simulink model "Buck_DCM_Due"  (R2020a)
settings: Solver=FixedStepAuto  StartTime=0.0  StopTime=10  FixedStep=T  RelTol=1e-3  EnableMultiTasking=on
undefined symbols (not defined in the file): C, ILmax, Iumax, J, Ki_I, Ki_IL, Kp_I, Kp_IL, Kp_Uc, Kp_W, Kphi, L, Lu, rL, Ru, T, Ubat, Ucmax, wmax
libraries: arduinolib x20, simulink x16
(part 1 of 2)
settings Model: SILPILModeSetting=veronly  ExtModeTrigDuration=2  Creator=Nguyen Tung  LastModifiedBy=Nguyen Tung
settings SolverCC: PositivePriorityOrder=on
settings OptimizationCC: StrengthReduction=on  PassReuseOutputArgsAs=Individual arguments  ZeroExternalMemoryAtStartup=off  ZeroInternalMemoryAtStartup=off  MaxStackSize=64  OptimizeBlockOrder=speed  OptimizationPriority=Speed  OptimizationCustomize=off  MultiThreadedLoops=on  EfficientTunableParamExpr=on
settings DebuggingCC: ParameterTunabilityLossMsg=error
settings HardwareCC: ProdBitPerPointer=32  ProdBitPerSizeT=32  ProdBitPerPtrDiffT=32  ProdLargestAtomicInteger=Long  ProdLargestAtomicFloat=Double  ProdWordSize=32  ProdHWDeviceType=ARM Compatible->ARM Cortex
settings SFSimCC: MATLABDynamicMemAlloc=off
settings RTWCC: SystemTargetFile=ert.tlc  HardwareBoard=Arduino Due  TLCOptions="-aInlineSetEventsForThisBaseRateFcn=TLC_FALSE -aSuppressMultiTaskScheduler=TLC_FALSE   -aRateBasedStepFcn=1"  TemplateMakefile=ert_default_tmf  Toolchain=Arduino ARM  BuildConfiguration=Faster Runs
settings CodeAppCC: ForceParamTrailComments=on  IgnoreCustomStorageClasses=off  OperatorAnnotations=on  SimulinkDataObjDesc=on  SFDataObjDesc=on  InsertBlockDesc=on
settings ERTTargetCC: SupportContinuousTime=on  SupportVariableSizeSignals=on  ExtModeStaticAllocSize=24576

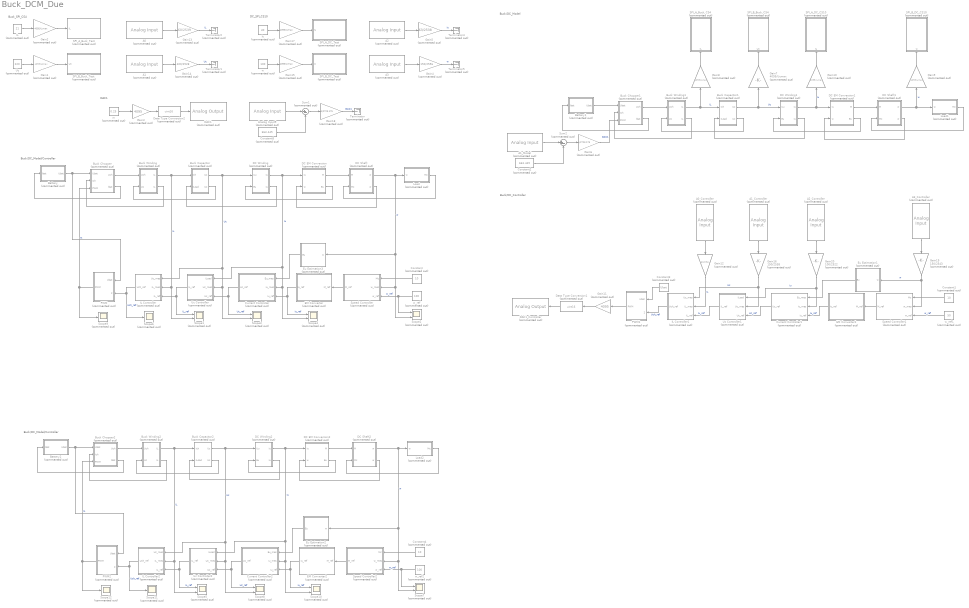
== system Buck_DCM_Due ==
  note: Buck/DC_Controller
  note: Buck/DC_Model
  note: Buck/DC_Model/Controller
  note: DAC1
  note: Buck_SPI_CS4
  note: DC_SPI_CS10
  note: Buck/DC_Model/Controller
  A0 : arduinolib/Analog Input  Commented=on  pinNumber=0  ReadResultsOnly=off  ConversionTriggerSource=Software  ExternalTriggerType=uint32( 0 )  OutputDataType=uint16  EnableConversionCompleteNotify=off  EnableOuputStatus=off  SampleTime=T  blockPlatform=arduino
  A0_Controller : arduinolib/Analog Input  Commented=on  pinNumber=0  ReadResultsOnly=off  ConversionTriggerSource=Software  ExternalTriggerType=uint32( 0 )  OutputDataType=uint16  EnableConversionCompleteNotify=off  EnableOuputStatus=off  SampleTime=T  blockPlatform=arduino
  A1 : arduinolib/Analog Input  Commented=on  pinNumber=1  ReadResultsOnly=off  ConversionTriggerSource=Software  ExternalTriggerType=uint32( 0 )  OutputDataType=uint16  EnableConversionCompleteNotify=off  EnableOuputStatus=off  SampleTime=T  blockPlatform=arduino
  A1_Controller : arduinolib/Analog Input  Commented=on  pinNumber=1  ReadResultsOnly=off  ConversionTriggerSource=Software  ExternalTriggerType=uint32( 0 )  OutputDataType=uint16  EnableConversionCompleteNotify=off  EnableOuputStatus=off  SampleTime=T  blockPlatform=arduino
  A1_Model : arduinolib/Analog Input  Commented=on  pinNumber=1  ReadResultsOnly=off  ConversionTriggerSource=Software  ExternalTriggerType=uint32( 0 )  OutputDataType=uint16  EnableConversionCompleteNotify=off  EnableOuputStatus=off  SampleTime=T  blockPlatform=arduino
  A2 : arduinolib/Analog Input  Commented=on  pinNumber=2  ReadResultsOnly=off  ConversionTriggerSource=Software  ExternalTriggerType=uint32( 0 )  OutputDataType=uint16  EnableConversionCompleteNotify=off  EnableOuputStatus=off  SampleTime=T  blockPlatform=arduino
  A2_Controller : arduinolib/Analog Input  Commented=on  pinNumber=2  ReadResultsOnly=off  ConversionTriggerSource=Software  ExternalTriggerType=uint32( 0 )  OutputDataType=uint16  EnableConversionCompleteNotify=off  EnableOuputStatus=off  SampleTime=T  blockPlatform=arduino
  A3 : arduinolib/Analog Input  Commented=on  pinNumber=3  ReadResultsOnly=off  ConversionTriggerSource=Software  ExternalTriggerType=uint32( 0 )  OutputDataType=uint16  EnableConversionCompleteNotify=off  EnableOuputStatus=off  SampleTime=T  blockPlatform=arduino
  A3_Controller : arduinolib/Analog Input  Commented=on  pinNumber=3  ReadResultsOnly=off  ConversionTriggerSource=Software  ExternalTriggerType=uint32( 0 )  OutputDataType=uint16  EnableConversionCompleteNotify=off  EnableOuputStatus=off  SampleTime=T  blockPlatform=arduino
  Analog Input9 : arduinolib/Analog Input  Commented=on  pinNumber=1  ReadResultsOnly=off  ConversionTriggerSource=Software  ExternalTriggerType=uint32( 0 )  OutputDataType=uint16  EnableConversionCompleteNotify=off  EnableOuputStatus=off  SampleTime=T  blockPlatform=arduino
  Battery : Subsystem  Commented=on  AncestorBlock=simulink/REM/SE
      mask Display:
      | plot(0,0,100,100, 1.2*[50,57.68,60.77,63.08,64.97,66.58,68,69.26,70.4, 	71.42,72.36,78.28,80,78.28,72.36,71.42,70.4, 	69.26,68,66.58,64.97,63.08,60.77,57.68,50,42.32, 	39.23,36.92,35.03,33.42,32,30.74,29.6,28.58, 	27.64,21.72,20,21.72,27.64,28.58,29.6,30.74,32, 	33.42,35.03,36.92,39.23,42.32,50]-10, 1.2*[20,21,22,23,24,25,26,27,28,29,30,40,50,60,70,71,72, 	73,74,75,76,77,78,79,80,79,78,77,76,75,74,73,72, 	71,70,60,50,40,30,29,28,27,26,25,24,23,22,21,20]-10)
      | disp('ES')
  Battery1 : Subsystem  Commented=on  AncestorBlock=simulink/REM/SE
      mask Display:
      | plot(0,0,100,100, 1.2*[50,57.68,60.77,63.08,64.97,66.58,68,69.26,70.4, 	71.42,72.36,78.28,80,78.28,72.36,71.42,70.4, 	69.26,68,66.58,64.97,63.08,60.77,57.68,50,42.32, 	39.23,36.92,35.03,33.42,32,30.74,29.6,28.58, 	27.64,21.72,20,21.72,27.64,28.58,29.6,30.74,32, 	33.42,35.03,36.92,39.23,42.32,50]-10, 1.2*[20,21,22,23,24,25,26,27,28,29,30,40,50,60,70,71,72, 	73,74,75,76,77,78,79,80,79,78,77,76,75,74,73,72, 	71,70,60,50,40,30,29,28,27,26,25,24,23,22,21,20]-10)
      | disp('ES')
  Battery2 : Subsystem  Commented=on  AncestorBlock=simulink/REM/SE
      mask Display:
      | plot(0,0,100,100, 1.2*[50,57.68,60.77,63.08,64.97,66.58,68,69.26,70.4, 	71.42,72.36,78.28,80,78.28,72.36,71.42,70.4, 	69.26,68,66.58,64.97,63.08,60.77,57.68,50,42.32, 	39.23,36.92,35.03,33.42,32,30.74,29.6,28.58, 	27.64,21.72,20,21.72,27.64,28.58,29.6,30.74,32, 	33.42,35.03,36.92,39.23,42.32,50]-10, 1.2*[20,21,22,23,24,25,26,27,28,29,30,40,50,60,70,71,72, 	73,74,75,76,77,78,79,80,79,78,77,76,75,74,73,72, 	71,70,60,50,40,30,29,28,27,26,25,24,23,22,21,20]-10)
      | disp('ES')
  Buck Capacitor : Subsystem  Commented=on  AncestorBlock=simulink/REM/EA  mask(CM){}
      mask Display: plot(0,0,100,100,[10,10,90,90,10],[90,10,10,90,90], [10,90],[10,90])
  Buck Capacitor1 : Subsystem  Commented=on  AncestorBlock=simulink/REM/EA  mask(CM){}
      mask Display: plot(0,0,100,100,[10,10,90,90,10],[90,10,10,90,90], [10,90],[10,90])
  Buck Capacitor2 : Subsystem  Commented=on  AncestorBlock=simulink/REM/EA  mask(CM){}
      mask Display: plot(0,0,100,100,[10,10,90,90,10],[90,10,10,90,90], [10,90],[10,90])
  Buck Chopper : Subsystem  Commented=on  AncestorBlock=simulink/REM/EC Elec  mask(Hacheur){}
      mask Display: plot(0,0,100,100,[10,10,90,90,10],[90,10,10,90,90])
  Buck Chopper1 : Subsystem  Commented=on  AncestorBlock=simulink/REM/EC Elec  mask(Hacheur){}
      mask Display: plot(0,0,100,100,[10,10,90,90,10],[90,10,10,90,90])
  Buck Chopper2 : Subsystem  Commented=on  AncestorBlock=simulink/REM/EC Elec  mask(Hacheur){}
      mask Display: plot(0,0,100,100,[10,10,90,90,10],[90,10,10,90,90])
  Buck Winding : Subsystem  Commented=on  AncestorBlock=simulink/REM/EA  mask(CM){}
      mask Display: plot(0,0,100,100,[10,10,90,90,10],[90,10,10,90,90], [10,90],[10,90])
  Buck Winding1 : Subsystem  Commented=on  AncestorBlock=simulink/REM/EA  mask(CM){}
      mask Display: plot(0,0,100,100,[10,10,90,90,10],[90,10,10,90,90], [10,90],[10,90])
  Buck Winding2 : Subsystem  Commented=on  AncestorBlock=simulink/REM/EA  mask(CM){}
      mask Display: plot(0,0,100,100,[10,10,90,90,10],[90,10,10,90,90], [10,90],[10,90])
  Constant : Constant  Commented=on  Value=10
  Constant1 : Constant  Commented=on  Value=10
  Constant2 : Constant  Commented=on  Value=663.445
  Constant3 : Constant  Commented=on  Value=Ubat
  Constant4 : Constant  Commented=on  Value=10
  Constant8 : Constant  Commented=on  Value=663.445
  Current Controller : Subsystem  Commented=on  AncestorBlock=simulink/SMC/Asservissement Correcteur IP
      mask Display: plot(0,0,100,100, [10,30,90,70,10,90],[90,10,10,90,90,10])
  Current Controller1 : Subsystem  Commented=on  AncestorBlock=simulink/SMC/Asservissement Correcteur IP
      mask Display: plot(0,0,100,100, [10,30,90,70,10,90],[90,10,10,90,90,10])
  Current Controller2 : Subsystem  Commented=on  AncestorBlock=simulink/SMC/Asservissement Correcteur IP
      mask Display: plot(0,0,100,100, [10,30,90,70,10,90],[90,10,10,90,90,10])
  DAC1 : arduinolib/Analog Output  Commented=on  DACpin=DAC1  blockPlatform=arduino
      settings: SourceProductBaseCode=ARDUINO
  DAC1_Controller : arduinolib/Analog Output  Commented=on  DACpin=DAC1  blockPlatform=arduino
      settings: SourceProductBaseCode=ARDUINO
  DC EM Conversion : Subsystem  Commented=on  AncestorBlock=simulink/REM/EC EM
      mask Display: plot(0,0,100,100, 1.4*[50,57.68,60.77,63.08,64.97,66.58,68,69.26,70.4, 	71.42,72.36,78.28,80,78.28,72.36,71.42,70.4, 	69.26,68,66.58,64.97,63.08,60.77,57.68,50,42.32, 	39.23,36.92,35.03,33.42,32,30.74,29.6,28.58, 	27.64,21.72,20,21.72,27.64,28.58,29.6,30.74,32, 	33.42,35.03,36.92,39.23,42.32,50]-20, 1.4*[20,21,22,23,24,25,26,27,28,29,30,40,50,60,70,71,72, 	73,74,75,76,77,78,79,80,79,78,77,76,75,74,73,72, 	71,70,60,50,40,30,29,28,27,26,25,24,23,22,21,20]-20)
  DC EM Conversion1 : Subsystem  Commented=on  AncestorBlock=simulink/REM/EC EM
      mask Display: plot(0,0,100,100, 1.4*[50,57.68,60.77,63.08,64.97,66.58,68,69.26,70.4, 	71.42,72.36,78.28,80,78.28,72.36,71.42,70.4, 	69.26,68,66.58,64.97,63.08,60.77,57.68,50,42.32, 	39.23,36.92,35.03,33.42,32,30.74,29.6,28.58, 	27.64,21.72,20,21.72,27.64,28.58,29.6,30.74,32, 	33.42,35.03,36.92,39.23,42.32,50]-20, 1.4*[20,21,22,23,24,25,26,27,28,29,30,40,50,60,70,71,72, 	73,74,75,76,77,78,79,80,79,78,77,76,75,74,73,72, 	71,70,60,50,40,30,29,28,27,26,25,24,23,22,21,20]-20)
  DC EM Conversion2 : Subsystem  Commented=on  AncestorBlock=simulink/REM/EC EM
      mask Display: plot(0,0,100,100, 1.4*[50,57.68,60.77,63.08,64.97,66.58,68,69.26,70.4, 	71.42,72.36,78.28,80,78.28,72.36,71.42,70.4, 	69.26,68,66.58,64.97,63.08,60.77,57.68,50,42.32, 	39.23,36.92,35.03,33.42,32,30.74,29.6,28.58, 	27.64,21.72,20,21.72,27.64,28.58,29.6,30.74,32, 	33.42,35.03,36.92,39.23,42.32,50]-20, 1.4*[20,21,22,23,24,25,26,27,28,29,30,40,50,60,70,71,72, 	73,74,75,76,77,78,79,80,79,78,77,76,75,74,73,72, 	71,70,60,50,40,30,29,28,27,26,25,24,23,22,21,20]-20)
  DC Shaft : Subsystem  Commented=on  AncestorBlock=simulink/REM/EA  mask(CM){}
      mask Display: plot(0,0,100,100,[10,10,90,90,10],[90,10,10,90,90], [10,90],[10,90])
  DC Shaft1 : Subsystem  Commented=on  AncestorBlock=simulink/REM/EA  mask(CM){}
      mask Display: plot(0,0,100,100,[10,10,90,90,10],[90,10,10,90,90], [10,90],[10,90])
  DC Shaft2 : Subsystem  Commented=on  AncestorBlock=simulink/REM/EA  mask(CM){}
      mask Display: plot(0,0,100,100,[10,10,90,90,10],[90,10,10,90,90], [10,90],[10,90])
  DC Winding : Subsystem  Commented=on  AncestorBlock=simulink/REM/EA  mask(CM){}
      mask Display: plot(0,0,100,100,[10,10,90,90,10],[90,10,10,90,90], [10,90],[10,90])
  DC Winding1 : Subsystem  Commented=on  AncestorBlock=simulink/REM/EA  mask(CM){}
      mask Display: plot(0,0,100,100,[10,10,90,90,10],[90,10,10,90,90], [10,90],[10,90])
  DC Winding2 : Subsystem  Commented=on  AncestorBlock=simulink/REM/EA  mask(CM){}
      mask Display: plot(0,0,100,100,[10,10,90,90,10],[90,10,10,90,90], [10,90],[10,90])
  Data Type Conversion1 : DataTypeConversion  Commented=on  OutDataTypeStr=uint16  RndMeth=Nearest
  Data Type Conversion2 : DataTypeConversion  Commented=on  OutDataTypeStr=uint16  RndMeth=Nearest
  EM Converter : Subsystem  Commented=on  AncestorBlock=simulink/SMC/Inversion EC avec mesure
      mask Display: plot(0,0,100,100,[10,30,90,70,10],[90,10,10,90,90])
  EM Converter1 : Subsystem  Commented=on  AncestorBlock=simulink/SMC/Inversion EC avec mesure
      mask Display: plot(0,0,100,100,[10,30,90,70,10],[90,10,10,90,90])
  EM Converter2 : Subsystem  Commented=on  AncestorBlock=simulink/SMC/Inversion EC avec mesure
      mask Display: plot(0,0,100,100,[10,30,90,70,10],[90,10,10,90,90])
  Eu Estimation1 : Subsystem  Commented=on  AncestorBlock=simulink/REM/EC EM
      mask Display: plot(0,0,100,100, 1.4*[50,57.68,60.77,63.08,64.97,66.58,68,69.26,70.4, 	71.42,72.36,78.28,80,78.28,72.36,71.42,70.4, 	69.26,68,66.58,64.97,63.08,60.77,57.68,50,42.32, 	39.23,36.92,35.03,33.42,32,30.74,29.6,28.58, 	27.64,21.72,20,21.72,27.64,28.58,29.6,30.74,32, 	33.42,35.03,36.92,39.23,42.32,50]-20, 1.4*[20,21,22,23,24,25,26,27,28,29,30,40,50,60,70,71,72, 	73,74,75,76,77,78,79,80,79,78,77,76,75,74,73,72, 	71,70,60,50,40,30,29,28,27,26,25,24,23,22,21,20]-20)
  Eu Estimation2 : Subsystem  Commented=on  AncestorBlock=simulink/REM/EC EM
      mask Display: plot(0,0,100,100, 1.4*[50,57.68,60.77,63.08,64.97,66.58,68,69.26,70.4, 	71.42,72.36,78.28,80,78.28,72.36,71.42,70.4, 	69.26,68,66.58,64.97,63.08,60.77,57.68,50,42.32, 	39.23,36.92,35.03,33.42,32,30.74,29.6,28.58, 	27.64,21.72,20,21.72,27.64,28.58,29.6,30.74,32, 	33.42,35.03,36.92,39.23,42.32,50]-20, 1.4*[20,21,22,23,24,25,26,27,28,29,30,40,50,60,70,71,72, 	73,74,75,76,77,78,79,80,79,78,77,76,75,74,73,72, 	71,70,60,50,40,30,29,28,27,26,25,24,23,22,21,20]-20)
  Eu Estimation3 : Subsystem  Commented=on  AncestorBlock=simulink/REM/EC EM
      mask Display: plot(0,0,100,100, 1.4*[50,57.68,60.77,63.08,64.97,66.58,68,69.26,70.4, 	71.42,72.36,78.28,80,78.28,72.36,71.42,70.4, 	69.26,68,66.58,64.97,63.08,60.77,57.68,50,42.32, 	39.23,36.92,35.03,33.42,32,30.74,29.6,28.58, 	27.64,21.72,20,21.72,27.64,28.58,29.6,30.74,32, 	33.42,35.03,36.92,39.23,42.32,50]-20, 1.4*[20,21,22,23,24,25,26,27,28,29,30,40,50,60,70,71,72, 	73,74,75,76,77,78,79,80,79,78,77,76,75,74,73,72, 	71,70,60,50,40,30,29,28,27,26,25,24,23,22,21,20]-20)
  Gain1 : Gain  Commented=on  Gain=4095/Ucmax
  Gain10 : Gain  Commented=on  Gain=4095/Iumax
  Gain11 : Gain  Commented=on  Gain=4095
  Gain12 : Gain  Commented=on  Gain=60/2541
  Gain13 : Gain  Commented=on  Gain=60/2539
  Gain14 : Gain  Commented=on  Gain=400/2528
  Gain15 : Gain  Commented=on  Gain=4095/wmax
  Gain16 : Gain  Commented=on  Gain=150/2538
  Gain17 : Gain  Commented=on  Gain=4095/Iumax
  Gain18 : Gain  Commented=on  Gain=1/2723.175
  Gain19 : Gain  Commented=on  Gain=150/2543
  Gain2 : Gain  Commented=on  Gain=4095/ILmax
  Gain20 : Gain  Commented=on  Gain=100/2522
  Gain3 : Gain  Commented=on  Gain=4095
  Gain4 : Gain  Commented=on  Gain=150/2556
  Gain5 : Gain  Commented=on  Gain=63/2538
  Gain6 : Gain  Commented=on  Gain=1/2723.175
  Gain7 : Gain  Commented=on  Gain=4095/Ucmax
  Gain8 : Gain  Commented=on  Gain=4095/ILmax
  Gain9 : Gain  Commented=on  Gain=4095/wmax
  IL : Constant  Commented=on  Value=21
  IL Controller : Subsystem  Commented=on  AncestorBlock=simulink/SMC/Asservissement Correcteur IP
      mask Display: plot(0,0,100,100, [10,30,90,70,10,90],[90,10,10,90,90,10])
  IL Controller1 : Subsystem  Commented=on  AncestorBlock=simulink/SMC/Asservissement Correcteur IP
      mask Display: plot(0,0,100,100, [10,30,90,70,10,90],[90,10,10,90,90,10])
  IL Controller2 : Subsystem  Commented=on  AncestorBlock=simulink/SMC/Asservissement Correcteur IP
      mask Display: plot(0,0,100,100, [10,30,90,70,10,90],[90,10,10,90,90,10])
  Iu : Constant  Commented=on  Value=30  SampleTime=T
  Load : Subsystem  Commented=on  AncestorBlock=simulink/REM/SE
      mask Display:
      | plot(0,0,100,100, 1.2*[50,57.68,60.77,63.08,64.97,66.58,68,69.26,70.4, 	71.42,72.36,78.28,80,78.28,72.36,71.42,70.4, 	69.26,68,66.58,64.97,63.08,60.77,57.68,50,42.32, 	39.23,36.92,35.03,33.42,32,30.74,29.6,28.58, 	27.64,21.72,20,21.72,27.64,28.58,29.6,30.74,32, 	33.42,35.03,36.92,39.23,42.32,50]-10, 1.2*[20,21,22,23,24,25,26,27,28,29,30,40,50,60,70,71,72, 	73,74,75,76,77,78,79,80,79,78,77,76,75,74,73,72, 	71,70,60,50,40,30,29,28,27,26,25,24,23,22,21,20]-10)
      | disp('MS')
  Load1 : Subsystem  Commented=on  AncestorBlock=simulink/REM/SE
      mask Display:
      | plot(0,0,100,100, 1.2*[50,57.68,60.77,63.08,64.97,66.58,68,69.26,70.4, 	71.42,72.36,78.28,80,78.28,72.36,71.42,70.4, 	69.26,68,66.58,64.97,63.08,60.77,57.68,50,42.32, 	39.23,36.92,35.03,33.42,32,30.74,29.6,28.58, 	27.64,21.72,20,21.72,27.64,28.58,29.6,30.74,32, 	33.42,35.03,36.92,39.23,42.32,50]-10, 1.2*[20,21,22,23,24,25,26,27,28,29,30,40,50,60,70,71,72, 	73,74,75,76,77,78,79,80,79,78,77,76,75,74,73,72, 	71,70,60,50,40,30,29,28,27,26,25,24,23,22,21,20]-10)
      | disp('MS')
  Load2 : Subsystem  Commented=on  AncestorBlock=simulink/REM/SE
      mask Display:
      | plot(0,0,100,100, 1.2*[50,57.68,60.77,63.08,64.97,66.58,68,69.26,70.4, 	71.42,72.36,78.28,80,78.28,72.36,71.42,70.4, 	69.26,68,66.58,64.97,63.08,60.77,57.68,50,42.32, 	39.23,36.92,35.03,33.42,32,30.74,29.6,28.58, 	27.64,21.72,20,21.72,27.64,28.58,29.6,30.74,32, 	33.42,35.03,36.92,39.23,42.32,50]-10, 1.2*[20,21,22,23,24,25,26,27,28,29,30,40,50,60,70,71,72, 	73,74,75,76,77,78,79,80,79,78,77,76,75,74,73,72, 	71,70,60,50,40,30,29,28,27,26,25,24,23,22,21,20]-10)
      | disp('MS')
  PWM : Subsystem  Commented=on  AncestorBlock=simulink/SMC/Inversion EC avec mesure
      mask Display: plot(0,0,100,100,[10,30,90,70,10],[90,10,10,90,90])
  PWM1 : Subsystem  Commented=on  AncestorBlock=simulink/SMC/Inversion EC avec mesure
      mask Display: plot(0,0,100,100,[10,30,90,70,10],[90,10,10,90,90])
  PWM2 : Subsystem  Commented=on  AncestorBlock=simulink/SMC/Inversion EC avec mesure
      mask Display: plot(0,0,100,100,[10,30,90,70,10],[90,10,10,90,90])
  SPI_A_Buck_CS4 : Subsystem  Commented=on
  SPI_A_Buck_Test : Subsystem  Commented=on
  SPI_A_DC_CS10 : Subsystem  Commented=on
  SPI_A_DC_Test : Subsystem  Commented=on
  SPI_B_Buck_CS4 : Subsystem  Commented=on
  SPI_B_Buck_Test : Subsystem  Commented=on
  SPI_B_DC_CS10 : Subsystem  Commented=on
  SPI_B_DC_Test : Subsystem  Commented=on
  Scope{1..5,7..8,10} (8 alike) : Scope  Commented=on  NumInputPorts=2
  Scope{6,9,11..12} (4 alike) : Scope  Commented=on
  Speed Controller : Subsystem  Commented=on  AncestorBlock=simulink/SMC/Asservissement Correcteur IP
      mask Display: plot(0,0,100,100, [10,30,90,70,10,90],[90,10,10,90,90,10])
  Speed Controller1 : Subsystem  Commented=on  AncestorBlock=simulink/SMC/Asservissement Correcteur IP
      mask Display: plot(0,0,100,100, [10,30,90,70,10,90],[90,10,10,90,90,10])
  Speed Controller2 : Subsystem  Commented=on  AncestorBlock=simulink/SMC/Asservissement Correcteur IP
      mask Display: plot(0,0,100,100, [10,30,90,70,10,90],[90,10,10,90,90,10])
  Sum1 : Sum  Commented=on  Inputs=|+-
  Sum2 : Sum  Commented=on  Inputs=|+-
  Terminator{,1..2,4..5} (5 alike) : Terminator  Commented=on
  Uc : Constant  Commented=on  Value=220
  Uc Controller : Subsystem  Commented=on  AncestorBlock=simulink/SMC/Asservissement Correcteur IP
      mask Display: plot(0,0,100,100, [10,30,90,70,10,90],[90,10,10,90,90,10])
  Uc Controller1 : Subsystem  Commented=on  AncestorBlock=simulink/SMC/Asservissement Correcteur IP
      mask Display: plot(0,0,100,100, [10,30,90,70,10,90],[90,10,10,90,90,10])
  Uc Controller2 : Subsystem  Commented=on  AncestorBlock=simulink/SMC/Asservissement Correcteur IP
      mask Display: plot(0,0,100,100, [10,30,90,70,10,90],[90,10,10,90,90,10])
  m : Constant  Commented=on  Value=0.25
  w : Constant  Commented=on  Value=100  SampleTime=T
  w_ref : Constant  Commented=on  Value=100
  w_ref1 : Constant  Commented=on  Value=50
  w_ref2 : Constant  Commented=on  Value=100
  wires:
  m/1 -> Gain3/1
  Gain14/1 -> Terminator1/1  "Uc"
  A1/1 -> Gain14/1
  Constant8/1 -> Sum1/2
  Gain1/1 -> SPI_B_Buck_Test/1(Uc)
  IL/1 -> Gain2/1
  Data Type Conversion2/1 -> DAC1/1
  Gain13/1 -> Terminator2/1  "IL"
  A0/1 -> Gain13/1
  Gain3/1 -> Data Type Conversion2/1
  Gain18/1 -> Terminator/1  "DAC1"
  Analog Input9/1 -> Sum1/1
  Sum1/1 -> Gain18/1
  Uc/1 -> Gain1/1
  Gain2/1 -> SPI_A_Buck_Test/1(IL)
  Gain15/1 -> SPI_B_DC_Test/1(w)
  w/1 -> Gain15/1
  A3/1 -> Gain4/1
  Gain4/1 -> Terminator5/1  "w"
  Gain17/1 -> SPI_A_DC_Test/1(Iu)
  Iu/1 -> Gain17/1
  Gain5/1 -> Terminator4/1  "Iu"
  A2/1 -> Gain5/1
  DC Shaft/1(w) -> Load/1(w), Scope2/2, Speed Controller/2(w_mes), Eu Estimation3/1(w)  "w"
  w_ref/1 -> Scope2/1, Speed Controller/3(w_ref)  "w_ref"
  EM Converter/1(Iu_ref) -> Scope4/1, Current Controller/3(Iu_ref)  "Iu_ref"
  Eu Estimation3/1(Eu) -> Current Controller/1(Eu_mes)
  DC Shaft/2("w ") -> DC EM Conversion/2(w)
  DC EM Conversion/2(Eu) -> DC Winding/2(Eu)
  DC Winding/1(Iu) -> DC EM Conversion/1(Iu), Uc Controller/1(ILoad), Scope4/2, Current Controller/2(Iu_mes)  "Iu"
  Current Controller/1(Uc_ref) -> Scope3/1, Uc Controller/3(Uc_ref)  "Uc_ref"
  DC EM Conversion/1(M) -> DC Shaft/1(M)
  Load/1(Mc) -> DC Shaft/2(Mc)
  Speed Controller/1(M_ref) -> EM Converter/1(M_ref)
  PWM/1(PWM) -> Buck Chopper/3(PWM), Scope9/1  "m"
  Buck Chopper/1(Uch) -> Buck Winding/1(Uch)
  Buck Winding/2("IL ") -> Buck Chopper/2(Ich)
  IL Controller/1(Uch_ref) -> Scope6/1, PWM/2(Uch_ref)  "Uch_ref"
  Uc Controller/1(IL_ref) -> Scope1/1, IL Controller/3(IL_ref)  "IL_ref"
  Buck Capacitor/2("Uc ") -> Buck Winding/2(Uc)
  Buck Chopper/2(Ibat) -> Battery/1(Ibat)
  Battery/1(Ubat) -> Buck Chopper/1(Ubat), PWM/1(Ubat)
  Buck Winding/1(IL) -> Buck Capacitor/1(Ich), Scope1/2, IL Controller/2(IL_mes)  "IL"
  Buck Capacitor/1(Uc) -> IL Controller/1(Uc_mes), Scope3/2, Uc Controller/2(Uc_mes), DC Winding/1(Uu)  "Uc"
  DC Winding/2("Iu ") -> Buck Capacitor/2(ILoad)
  DC Shaft1/2("w ") -> DC EM Conversion1/2(w)
  Eu Estimation1/1(Eu) -> Current Controller1/1(Eu_mes)
  Speed Controller1/1(M_ref) -> EM Converter1/1(M_ref)
  DC EM Conversion1/2(Eu) -> DC Winding1/2(Eu)
  DC EM Conversion1/1(M) -> DC Shaft1/1(M)
  Battery1/1(Ubat) -> Buck Chopper1/1(Ubat)
  w_ref1/1 -> Speed Controller1/3(w_ref)  "w_ref"
  Buck Chopper1/2(Ibat) -> Battery1/1(Ibat)
  Buck Capacitor1/2("Uc ") -> Buck Winding1/2(Uc)
  EM Converter1/1(Iu_ref) -> Current Controller1/3(Iu_ref)  "Iu_ref"
  IL Controller1/1(Uch_ref) -> PWM1/2(Uch_ref)  "Uch_ref"
  Uc Controller1/1(IL_ref) -> IL Controller1/3(IL_ref)  "IL_ref"
  Load1/1(Mc) -> DC Shaft1/2(Mc)
  DC Shaft1/1(w) -> Load1/1(w), Gain9/1  "w"
  Buck Chopper1/1(Uch) -> Buck Winding1/1(Uch)
  Buck Winding1/2("IL ") -> Buck Chopper1/2(Ich)
  DC Winding1/2("Iu ") -> Buck Capacitor1/2(ILoad)
  Current Controller1/1(Uc_ref) -> Uc Controller1/3(Uc_ref)  "Uc_ref"
  Constant1/1 -> Speed Controller1/1(Mc)
  Constant/1 -> Speed Controller/1(Mc)
  Sum2/1 -> Gain6/1
  A1_Model/1 -> Sum2/1
  Constant2/1 -> Sum2/2
  Gain6/1 -> Buck Chopper1/3(PWM)  "DAC1"
  Gain8/1 -> SPI_A_Buck_CS4/1(IL)
  Buck Winding1/1(IL) -> Buck Capacitor1/1(Ich), Gain8/1  "IL"
  Gain7/1 -> SPI_B_Buck_CS4/1(Uc)
  Buck Capacitor1/1(Uc) -> DC Winding1/1(Uu), Gain7/1  "Uc"
  Gain10/1 -> SPI_A_DC_CS10/1(Iu)
  DC Winding1/1(Iu) -> Gain10/1, DC EM Conversion1/1(Iu)  "Iu"
  Gain9/1 -> SPI_B_DC_CS10/1(w)
  Gain11/1 -> Data Type Conversion1/1
  PWM1/1(PWM) -> Gain11/1
  Data Type Conversion1/1 -> DAC1_Controller/1
  Constant3/1 -> PWM1/1(Ubat)
  A1_Controller/1 -> Gain16/1
  A0_Controller/1 -> Gain12/1
  Gain12/1 -> IL Controller1/2(IL_mes)  "IL"
  Gain16/1 -> IL Controller1/1(Uc_mes), Uc Controller1/2(Uc_mes)  "Uc"
  A3_Controller/1 -> Gain19/1
  A2_Controller/1 -> Gain20/1
  Gain20/1 -> Uc Controller1/1(ILoad), Current Controller1/2(Iu_mes)  "Iu"
  Gain19/1 -> Speed Controller1/2(w_mes), Eu Estimation1/1(w)  "w"
  Buck Winding2/1(IL) -> Buck Capacitor2/1(Ich), Scope5/2, IL Controller2/2(IL_mes)  "IL"
  PWM2/1(PWM) -> Scope12/1, Buck Chopper2/3(PWM)  "m"
  Battery2/1(Ubat) -> Buck Chopper2/1(Ubat), PWM2/1(Ubat)
  Buck Chopper2/1(Uch) -> Buck Winding2/1(Uch)
  Current Controller2/1(Uc_ref) -> Scope8/1, Uc Controller2/3(Uc_ref)  "Uc_ref"
  DC Shaft2/1(w) -> Load2/1(w), Scope7/2, Speed Controller2/2(w_mes), Eu Estimation2/1(w)  "w"
  DC Shaft2/2("w ") -> DC EM Conversion2/2(w)
  DC Winding2/2("Iu ") -> Buck Capacitor2/2(ILoad)
  DC EM Conversion2/1(M) -> DC Shaft2/1(M)
  w_ref2/1 -> Scope7/1, Speed Controller2/3(w_ref)  "w_ref"
  Buck Winding2/2("IL ") -> Buck Chopper2/2(Ich)
  Speed Controller2/1(M_ref) -> EM Converter2/1(M_ref)
  Buck Capacitor2/1(Uc) -> IL Controller2/1(Uc_mes), Scope8/2, Uc Controller2/2(Uc_mes), DC Winding2/1(Uu)  "Uc"
  Constant4/1 -> Speed Controller2/1(Mc)
  Eu Estimation2/1(Eu) -> Current Controller2/1(Eu_mes)
  Uc Controller2/1(IL_ref) -> Scope5/1, IL Controller2/3(IL_ref)  "IL_ref"
  IL Controller2/1(Uch_ref) -> Scope11/1, PWM2/2(Uch_ref)  "Uch_ref"
  DC Winding2/1(Iu) -> DC EM Conversion2/1(Iu), Uc Controller2/1(ILoad), Scope10/2, Current Controller2/2(Iu_mes)  "Iu"
  DC EM Conversion2/2(Eu) -> DC Winding2/2(Eu)
  Buck Chopper2/2(Ibat) -> Battery2/1(Ibat)
  Buck Capacitor2/2("Uc ") -> Buck Winding2/2(Uc)
  EM Converter2/1(Iu_ref) -> Scope10/1, Current Controller2/3(Iu_ref)  "Iu_ref"
  Load2/1(Mc) -> DC Shaft2/2(Mc)

== system Buck_DCM_Due/Battery ==
  Ibat : Inport
  Constant : Constant  Value=Ubat
  Terminator : Terminator
  Ubat : Outport  InitialOutput=0  VectorParamsAs1DForOutWhenUnconnected=off
  wires:
  Constant/1 -> Ubat/1
  Ibat/1 -> Terminator/1

== system Buck_DCM_Due/Battery1 ==
  Ibat : Inport
  Constant : Constant  Value=Ubat
  Terminator : Terminator
  Ubat : Outport  InitialOutput=0  VectorParamsAs1DForOutWhenUnconnected=off
  wires:
  Constant/1 -> Ubat/1
  Ibat/1 -> Terminator/1

== system Buck_DCM_Due/Battery2 ==
  Ibat : Inport
  Constant : Constant  Value=Ubat
  Terminator : Terminator
  Ubat : Outport  InitialOutput=0  VectorParamsAs1DForOutWhenUnconnected=off
  wires:
  Constant/1 -> Ubat/1
  Ibat/1 -> Terminator/1

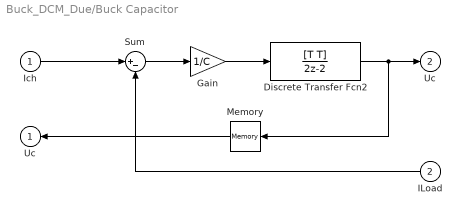
== system Buck_DCM_Due/Buck Capacitor ==
  Ich : Inport
  ILoad : Inport  Port=2
  Discrete Transfer Fcn2 : DiscreteTransferFcn  Numerator=[T T]  Denominator=[2 -2]
  Gain : Gain  Gain=1/C
  Memory : Memory
  Sum : Sum  Inputs=|+-
  Uc : Outport  InitialOutput=0  VectorParamsAs1DForOutWhenUnconnected=off
  "Uc " : Outport  Port=2  InitialOutput=0  VectorParamsAs1DForOutWhenUnconnected=off
  wires:
  Ich/1 -> Sum/1
  Sum/1 -> Gain/1
  Gain/1 -> Discrete Transfer Fcn2/1
  Discrete Transfer Fcn2/1 -> "Uc "/1, Memory/1
  ILoad/1 -> Sum/2
  Memory/1 -> Uc/1

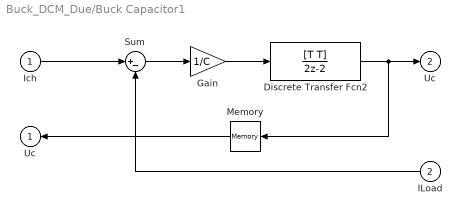
== system Buck_DCM_Due/Buck Capacitor1 ==
  Ich : Inport
  ILoad : Inport  Port=2
  Discrete Transfer Fcn2 : DiscreteTransferFcn  Numerator=[T T]  Denominator=[2 -2]
  Gain : Gain  Gain=1/C
  Memory : Memory
  Sum : Sum  Inputs=|+-
  Uc : Outport  InitialOutput=0  VectorParamsAs1DForOutWhenUnconnected=off
  "Uc " : Outport  Port=2  InitialOutput=0  VectorParamsAs1DForOutWhenUnconnected=off
  wires:
  Ich/1 -> Sum/1
  Sum/1 -> Gain/1
  Gain/1 -> Discrete Transfer Fcn2/1
  Discrete Transfer Fcn2/1 -> "Uc "/1, Memory/1
  ILoad/1 -> Sum/2
  Memory/1 -> Uc/1

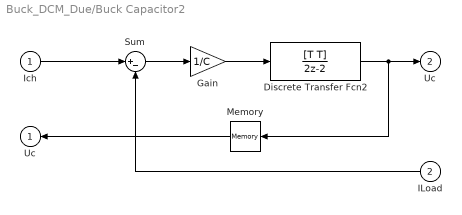
== system Buck_DCM_Due/Buck Capacitor2 ==
  Ich : Inport
  ILoad : Inport  Port=2
  Discrete Transfer Fcn2 : DiscreteTransferFcn  Numerator=[T T]  Denominator=[2 -2]
  Gain : Gain  Gain=1/C
  Memory : Memory
  Sum : Sum  Inputs=|+-
  Uc : Outport  InitialOutput=0  VectorParamsAs1DForOutWhenUnconnected=off
  "Uc " : Outport  Port=2  InitialOutput=0  VectorParamsAs1DForOutWhenUnconnected=off
  wires:
  Ich/1 -> Sum/1
  Sum/1 -> Gain/1
  Gain/1 -> Discrete Transfer Fcn2/1
  Discrete Transfer Fcn2/1 -> "Uc "/1, Memory/1
  ILoad/1 -> Sum/2
  Memory/1 -> Uc/1

== system Buck_DCM_Due/Buck Chopper ==
  Ubat : Inport
  Ich : Inport  Port=2
  PWM : Inport  Port=3
  Product : Product
  Product1 : Product
  Uch : Outport  InitialOutput=0  VectorParamsAs1DForOutWhenUnconnected=off
  Ibat : Outport  Port=2  InitialOutput=0  VectorParamsAs1DForOutWhenUnconnected=off
  wires:
  Product/1 -> Uch/1
  Ubat/1 -> Product/1
  PWM/1 -> Product1/2, Product/2
  Ich/1 -> Product1/1
  Product1/1 -> Ibat/1

== system Buck_DCM_Due/Buck Chopper1 ==
  Ubat : Inport
  Ich : Inport  Port=2
  PWM : Inport  Port=3
  Product : Product
  Product1 : Product
  Uch : Outport  InitialOutput=0  VectorParamsAs1DForOutWhenUnconnected=off
  Ibat : Outport  Port=2  InitialOutput=0  VectorParamsAs1DForOutWhenUnconnected=off
  wires:
  Product/1 -> Uch/1
  Ubat/1 -> Product/1
  PWM/1 -> Product1/2, Product/2
  Ich/1 -> Product1/1
  Product1/1 -> Ibat/1

== system Buck_DCM_Due/Buck Chopper2 ==
  Ubat : Inport
  Ich : Inport  Port=2
  PWM : Inport  Port=3
  Product : Product
  Product1 : Product
  Uch : Outport  InitialOutput=0  VectorParamsAs1DForOutWhenUnconnected=off
  Ibat : Outport  Port=2  InitialOutput=0  VectorParamsAs1DForOutWhenUnconnected=off
  wires:
  Product/1 -> Uch/1
  Ubat/1 -> Product/1
  PWM/1 -> Product1/2, Product/2
  Ich/1 -> Product1/1
  Product1/1 -> Ibat/1

== system Buck_DCM_Due/Buck Winding ==
  Uch : Inport
  Uc : Inport  Port=2
  Discrete Transfer Fcn : DiscreteTransferFcn  Numerator=[T T]  Denominator=[(2*L+rL*T) rL*T-2*L]
  Memory : Memory
  Sum : Sum  Inputs=|+-
  IL : Outport  InitialOutput=0  VectorParamsAs1DForOutWhenUnconnected=off
  "IL " : Outport  Port=2  InitialOutput=0  VectorParamsAs1DForOutWhenUnconnected=off
  wires:
  Uch/1 -> Sum/1
  Discrete Transfer Fcn/1 -> "IL "/1, Memory/1
  Sum/1 -> Discrete Transfer Fcn/1
  Uc/1 -> Sum/2
  Memory/1 -> IL/1

== system Buck_DCM_Due/Buck Winding1 ==
  Uch : Inport
  Uc : Inport  Port=2
  Discrete Transfer Fcn : DiscreteTransferFcn  Numerator=[T T]  Denominator=[(2*L+rL*T) rL*T-2*L]
  Memory : Memory
  Sum : Sum  Inputs=|+-
  IL : Outport  InitialOutput=0  VectorParamsAs1DForOutWhenUnconnected=off
  "IL " : Outport  Port=2  InitialOutput=0  VectorParamsAs1DForOutWhenUnconnected=off
  wires:
  Uch/1 -> Sum/1
  Discrete Transfer Fcn/1 -> "IL "/1, Memory/1
  Sum/1 -> Discrete Transfer Fcn/1
  Uc/1 -> Sum/2
  Memory/1 -> IL/1

== system Buck_DCM_Due/Buck Winding2 ==
  Uch : Inport
  Uc : Inport  Port=2
  Discrete Transfer Fcn : DiscreteTransferFcn  Numerator=[T T]  Denominator=[(2*L+rL*T) rL*T-2*L]
  Memory : Memory
  Sum : Sum  Inputs=|+-
  IL : Outport  InitialOutput=0  VectorParamsAs1DForOutWhenUnconnected=off
  "IL " : Outport  Port=2  InitialOutput=0  VectorParamsAs1DForOutWhenUnconnected=off
  wires:
  Uch/1 -> Sum/1
  Discrete Transfer Fcn/1 -> "IL "/1, Memory/1
  Sum/1 -> Discrete Transfer Fcn/1
  Uc/1 -> Sum/2
  Memory/1 -> IL/1

== system Buck_DCM_Due/Current Controller ==
  Eu_mes : Inport
  Iu_mes : Inport  Port=2
  Iu_ref : Inport  Port=3
  PI Controller : DiscreteTransferFcn  Numerator=[(2*Kp_I+Ki_I*T) -2*Kp_I+Ki_I*T]  Denominator=[2 -2]
  Saturation : Saturate  UpperLimit=Ubat  LowerLimit=0
  Sum : Sum  Inputs=|++
  Sum1 : Sum  Inputs=|-+
  Uc_ref : Outport  InitialOutput=0  VectorParamsAs1DForOutWhenUnconnected=off
  wires:
  Eu_mes/1 -> Sum/1
  Sum/1 -> Saturation/1
  Iu_mes/1 -> Sum1/1
  Sum1/1 -> PI Controller/1
  PI Controller/1 -> Sum/2
  Iu_ref/1 -> Sum1/2
  Saturation/1 -> Uc_ref/1

== system Buck_DCM_Due/Current Controller1 ==
  Eu_mes : Inport
  Iu_mes : Inport  Port=2
  Iu_ref : Inport  Port=3
  PI Controller : DiscreteTransferFcn  Numerator=[(2*Kp_I+Ki_I*T) -2*Kp_I+Ki_I*T]  Denominator=[2 -2]
  Saturation : Saturate  UpperLimit=Ubat  LowerLimit=0
  Sum : Sum  Inputs=|++
  Sum1 : Sum  Inputs=|-+
  Uc_ref : Outport  InitialOutput=0  VectorParamsAs1DForOutWhenUnconnected=off
  wires:
  Eu_mes/1 -> Sum/1
  Sum/1 -> Saturation/1
  Iu_mes/1 -> Sum1/1
  Sum1/1 -> PI Controller/1
  PI Controller/1 -> Sum/2
  Iu_ref/1 -> Sum1/2
  Saturation/1 -> Uc_ref/1

== system Buck_DCM_Due/Current Controller2 ==
  Eu_mes : Inport
  Iu_mes : Inport  Port=2
  Iu_ref : Inport  Port=3
  PI Controller : DiscreteTransferFcn  Numerator=[(2*Kp_I+Ki_I*T) -2*Kp_I+Ki_I*T]  Denominator=[2 -2]
  Saturation : Saturate  UpperLimit=Ubat  LowerLimit=0
  Sum : Sum  Inputs=|++
  Sum1 : Sum  Inputs=|-+
  Uc_ref : Outport  InitialOutput=0  VectorParamsAs1DForOutWhenUnconnected=off
  wires:
  Eu_mes/1 -> Sum/1
  Sum/1 -> Saturation/1
  Iu_mes/1 -> Sum1/1
  Sum1/1 -> PI Controller/1
  PI Controller/1 -> Sum/2
  Iu_ref/1 -> Sum1/2
  Saturation/1 -> Uc_ref/1

== system Buck_DCM_Due/DC EM Conversion ==
  Iu : Inport
  w : Inport  Port=2
  Gain : Gain  Gain=Kphi
  Gain1 : Gain  Gain=Kphi
  M : Outport  InitialOutput=0  VectorParamsAs1DForOutWhenUnconnected=off
  Eu : Outport  Port=2  InitialOutput=0  VectorParamsAs1DForOutWhenUnconnected=off
  wires:
  Iu/1 -> Gain/1
  Gain/1 -> M/1
  w/1 -> Gain1/1
  Gain1/1 -> Eu/1

== system Buck_DCM_Due/DC EM Conversion1 ==
  Iu : Inport
  w : Inport  Port=2
  Gain : Gain  Gain=Kphi
  Gain1 : Gain  Gain=Kphi
  M : Outport  InitialOutput=0  VectorParamsAs1DForOutWhenUnconnected=off
  Eu : Outport  Port=2  InitialOutput=0  VectorParamsAs1DForOutWhenUnconnected=off
  wires:
  Iu/1 -> Gain/1
  Gain/1 -> M/1
  w/1 -> Gain1/1
  Gain1/1 -> Eu/1

== system Buck_DCM_Due/DC EM Conversion2 ==
  Iu : Inport
  w : Inport  Port=2
  Gain : Gain  Gain=Kphi
  Gain1 : Gain  Gain=Kphi
  M : Outport  InitialOutput=0  VectorParamsAs1DForOutWhenUnconnected=off
  Eu : Outport  Port=2  InitialOutput=0  VectorParamsAs1DForOutWhenUnconnected=off
  wires:
  Iu/1 -> Gain/1
  Gain/1 -> M/1
  w/1 -> Gain1/1
  Gain1/1 -> Eu/1

== system Buck_DCM_Due/DC Shaft ==
  M : Inport
  Mc : Inport  Port=2
  Discrete Transfer Fcn2 : DiscreteTransferFcn  Numerator=[T T]  Denominator=[2 -2]
  Gain : Gain  Gain=1/J
  Memory : Memory
  Sum : Sum  Inputs=|+-
  w : Outport  InitialOutput=0  VectorParamsAs1DForOutWhenUnconnected=off
  "w " : Outport  Port=2  InitialOutput=0  VectorParamsAs1DForOutWhenUnconnected=off
  wires:
  M/1 -> Sum/1
  Mc/1 -> Sum/2
  Sum/1 -> Gain/1
  Discrete Transfer Fcn2/1 -> Memory/1, "w "/1
  Gain/1 -> Discrete Transfer Fcn2/1
  Memory/1 -> w/1

== system Buck_DCM_Due/DC Shaft1 ==
  M : Inport
  Mc : Inport  Port=2
  Discrete Transfer Fcn2 : DiscreteTransferFcn  Numerator=[T T]  Denominator=[2 -2]
  Gain : Gain  Gain=1/J
  Memory : Memory
  Sum : Sum  Inputs=|+-
  w : Outport  InitialOutput=0  VectorParamsAs1DForOutWhenUnconnected=off
  "w " : Outport  Port=2  InitialOutput=0  VectorParamsAs1DForOutWhenUnconnected=off
  wires:
  M/1 -> Sum/1
  Mc/1 -> Sum/2
  Sum/1 -> Gain/1
  Discrete Transfer Fcn2/1 -> Memory/1, "w "/1
  Gain/1 -> Discrete Transfer Fcn2/1
  Memory/1 -> w/1

== system Buck_DCM_Due/DC Shaft2 ==
  M : Inport
  Mc : Inport  Port=2
  Discrete Transfer Fcn2 : DiscreteTransferFcn  Numerator=[T T]  Denominator=[2 -2]
  Gain : Gain  Gain=1/J
  Memory : Memory
  Sum : Sum  Inputs=|+-
  w : Outport  InitialOutput=0  VectorParamsAs1DForOutWhenUnconnected=off
  "w " : Outport  Port=2  InitialOutput=0  VectorParamsAs1DForOutWhenUnconnected=off
  wires:
  M/1 -> Sum/1
  Mc/1 -> Sum/2
  Sum/1 -> Gain/1
  Discrete Transfer Fcn2/1 -> Memory/1, "w "/1
  Gain/1 -> Discrete Transfer Fcn2/1
  Memory/1 -> w/1

== system Buck_DCM_Due/DC Winding ==
  Uu : Inport
  Eu : Inport  Port=2
  Discrete Transfer Fcn : DiscreteTransferFcn  Numerator=[T T]  Denominator=[(2*Lu+Ru*T) Ru*T-2*Lu]
  Memory : Memory
  Sum : Sum  Inputs=|+-
  Iu : Outport  InitialOutput=0  VectorParamsAs1DForOutWhenUnconnected=off
  "Iu " : Outport  Port=2  InitialOutput=0  VectorParamsAs1DForOutWhenUnconnected=off
  wires:
  Uu/1 -> Sum/1
  Sum/1 -> Discrete Transfer Fcn/1
  Discrete Transfer Fcn/1 -> Memory/1, "Iu "/1
  Eu/1 -> Sum/2
  Memory/1 -> Iu/1

== system Buck_DCM_Due/DC Winding1 ==
  Uu : Inport
  Eu : Inport  Port=2
  Discrete Transfer Fcn : DiscreteTransferFcn  Numerator=[T T]  Denominator=[(2*Lu+Ru*T) Ru*T-2*Lu]
  Memory : Memory
  Sum : Sum  Inputs=|+-
  Iu : Outport  InitialOutput=0  VectorParamsAs1DForOutWhenUnconnected=off
  "Iu " : Outport  Port=2  InitialOutput=0  VectorParamsAs1DForOutWhenUnconnected=off
  wires:
  Uu/1 -> Sum/1
  Sum/1 -> Discrete Transfer Fcn/1
  Discrete Transfer Fcn/1 -> Memory/1, "Iu "/1
  Eu/1 -> Sum/2
  Memory/1 -> Iu/1

== system Buck_DCM_Due/DC Winding2 ==
  Uu : Inport
  Eu : Inport  Port=2
  Discrete Transfer Fcn : DiscreteTransferFcn  Numerator=[T T]  Denominator=[(2*Lu+Ru*T) Ru*T-2*Lu]
  Memory : Memory
  Sum : Sum  Inputs=|+-
  Iu : Outport  InitialOutput=0  VectorParamsAs1DForOutWhenUnconnected=off
  "Iu " : Outport  Port=2  InitialOutput=0  VectorParamsAs1DForOutWhenUnconnected=off
  wires:
  Uu/1 -> Sum/1
  Sum/1 -> Discrete Transfer Fcn/1
  Discrete Transfer Fcn/1 -> Memory/1, "Iu "/1
  Eu/1 -> Sum/2
  Memory/1 -> Iu/1

== system Buck_DCM_Due/EM Converter ==
  M_ref : Inport
  Gain : Gain  Gain=1/Kphi
  Saturation : Saturate  UpperLimit=Iumax  LowerLimit=0
  Iu_ref : Outport  InitialOutput=0  VectorParamsAs1DForOutWhenUnconnected=off
  wires:
  M_ref/1 -> Gain/1
  Gain/1 -> Saturation/1
  Saturation/1 -> Iu_ref/1

== system Buck_DCM_Due/EM Converter1 ==
  M_ref : Inport
  Gain : Gain  Gain=1/Kphi
  Saturation : Saturate  UpperLimit=Iumax  LowerLimit=0
  Iu_ref : Outport  InitialOutput=0  VectorParamsAs1DForOutWhenUnconnected=off
  wires:
  M_ref/1 -> Gain/1
  Gain/1 -> Saturation/1
  Saturation/1 -> Iu_ref/1

== system Buck_DCM_Due/EM Converter2 ==
  M_ref : Inport
  Gain : Gain  Gain=1/Kphi
  Saturation : Saturate  UpperLimit=Iumax  LowerLimit=0
  Iu_ref : Outport  InitialOutput=0  VectorParamsAs1DForOutWhenUnconnected=off
  wires:
  M_ref/1 -> Gain/1
  Gain/1 -> Saturation/1
  Saturation/1 -> Iu_ref/1

== system Buck_DCM_Due/Eu Estimation1 ==
  w : Inport
  Gain1 : Gain  Gain=Kphi
  Eu : Outport  InitialOutput=0  VectorParamsAs1DForOutWhenUnconnected=off
  wires:
  w/1 -> Gain1/1
  Gain1/1 -> Eu/1

== system Buck_DCM_Due/Eu Estimation2 ==
  w : Inport
  Gain1 : Gain  Gain=Kphi
  Eu : Outport  InitialOutput=0  VectorParamsAs1DForOutWhenUnconnected=off
  wires:
  w/1 -> Gain1/1
  Gain1/1 -> Eu/1

== system Buck_DCM_Due/Eu Estimation3 ==
  w : Inport
  Gain1 : Gain  Gain=Kphi
  Eu : Outport  InitialOutput=0  VectorParamsAs1DForOutWhenUnconnected=off
  wires:
  w/1 -> Gain1/1
  Gain1/1 -> Eu/1

== system Buck_DCM_Due/IL Controller ==
  Uc_mes : Inport
  IL_mes : Inport  Port=2
  IL_ref : Inport  Port=3
  PI Controller : DiscreteTransferFcn  Numerator=[(2*Kp_IL+Ki_IL*T) -2*Kp_IL+Ki_IL*T]  Denominator=[2 -2]
  Saturation : Saturate  UpperLimit=Ubat  LowerLimit=0
  Sum : Sum  Inputs=++|
  Sum1 : Sum  Inputs=|-+
  Uch_ref : Outport  InitialOutput=0
  wires:
  Uc_mes/1 -> Sum/1
  IL_ref/1 -> Sum1/2
  IL_mes/1 -> Sum1/1
  Sum/1 -> Saturation/1
  Saturation/1 -> Uch_ref/1
  PI Controller/1 -> Sum/2
  Sum1/1 -> PI Controller/1

== system Buck_DCM_Due/IL Controller1 ==
  Uc_mes : Inport
  IL_mes : Inport  Port=2
  IL_ref : Inport  Port=3
  PI Controller : DiscreteTransferFcn  Numerator=[(2*Kp_IL+Ki_IL*T) -2*Kp_IL+Ki_IL*T]  Denominator=[2 -2]
  Saturation : Saturate  UpperLimit=Ubat  LowerLimit=0
  Sum : Sum  Inputs=++|
  Sum1 : Sum  Inputs=|-+
  Uch_ref : Outport  InitialOutput=0
  wires:
  Uc_mes/1 -> Sum/1
  IL_ref/1 -> Sum1/2
  IL_mes/1 -> Sum1/1
  Sum/1 -> Saturation/1
  Saturation/1 -> Uch_ref/1
  PI Controller/1 -> Sum/2
  Sum1/1 -> PI Controller/1

== system Buck_DCM_Due/IL Controller2 ==
  Uc_mes : Inport
  IL_mes : Inport  Port=2
  IL_ref : Inport  Port=3
  PI Controller : DiscreteTransferFcn  Numerator=[(2*Kp_IL+Ki_IL*T) -2*Kp_IL+Ki_IL*T]  Denominator=[2 -2]
  Saturation : Saturate  UpperLimit=Ubat  LowerLimit=0
  Sum : Sum  Inputs=++|
  Sum1 : Sum  Inputs=|-+
  Uch_ref : Outport  InitialOutput=0
  wires:
  Uc_mes/1 -> Sum/1
  IL_ref/1 -> Sum1/2
  IL_mes/1 -> Sum1/1
  Sum/1 -> Saturation/1
  Saturation/1 -> Uch_ref/1
  PI Controller/1 -> Sum/2
  Sum1/1 -> PI Controller/1

== system Buck_DCM_Due/Load ==
  w : Inport
  Load : Step  Time=5  After=10  SampleTime=T
  Terminator : Terminator
  Mc : Outport  InitialOutput=0  VectorParamsAs1DForOutWhenUnconnected=off
  wires:
  w/1 -> Terminator/1
  Load/1 -> Mc/1

== system Buck_DCM_Due/Load1 ==
  w : Inport
  Load : Step  Time=5  After=10  SampleTime=T
  Terminator : Terminator
  Mc : Outport  InitialOutput=0  VectorParamsAs1DForOutWhenUnconnected=off
  wires:
  w/1 -> Terminator/1
  Load/1 -> Mc/1

== system Buck_DCM_Due/Load2 ==
  w : Inport
  Load : Step  Time=5  After=10  SampleTime=T
  Terminator : Terminator
  Mc : Outport  InitialOutput=0  VectorParamsAs1DForOutWhenUnconnected=off
  wires:
  w/1 -> Terminator/1
  Load/1 -> Mc/1

== system Buck_DCM_Due/PWM ==
  Ubat : Inport
  Uch_ref : Inport  Port=2
  Divide : Product  Inputs=/*
  PWM : Outport
  wires:
  Divide/1 -> PWM/1
  Ubat/1 -> Divide/1
  Uch_ref/1 -> Divide/2

== system Buck_DCM_Due/PWM1 ==
  Ubat : Inport
  Uch_ref : Inport  Port=2
  Divide : Product  Inputs=/*
  PWM : Outport
  wires:
  Divide/1 -> PWM/1
  Ubat/1 -> Divide/1
  Uch_ref/1 -> Divide/2

== system Buck_DCM_Due/PWM2 ==
  Ubat : Inport
  Uch_ref : Inport  Port=2
  Divide : Product  Inputs=/*
  PWM : Outport
  wires:
  Divide/1 -> PWM/1
  Ubat/1 -> Divide/1
  Uch_ref/1 -> Divide/2

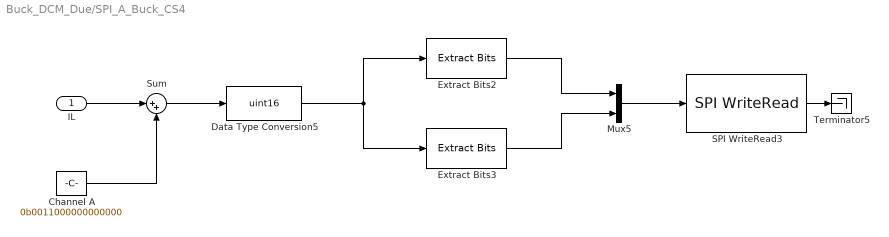
== system Buck_DCM_Due/SPI_A_Buck_CS4 ==
  IL : Inport
  Channel A : Constant  Value=0b0011000000000000
  Data Type Conversion5 : DataTypeConversion  OutDataTypeStr=uint16  RndMeth=Nearest
  Extract Bits2 : simulink/Logic and Bit Operations/Extract Bits  bitsToExtract=Range starting with most significant bit  numBits=8  bitIdxRange=[0 7]  outScalingMode=Treat bit field as an integer
  Extract Bits3 : simulink/Logic and Bit Operations/Extract Bits  bitsToExtract=Range ending with least significant bit  numBits=8  bitIdxRange=[0 7]  outScalingMode=Treat bit field as an integer
  Mux5 : Mux  Inputs=2
  SPI WriteRead3 : arduinolib/SPI WriteRead  slaveSelectPin_=4  blockPlatform=arduino
      settings: SourceProductBaseCode=ARDUINO
  Sum : Sum  Inputs=|++
  Terminator5 : Terminator
  wires:
  Extract Bits3/1 -> Mux5/2
  Mux5/1 -> SPI WriteRead3/1
  Channel A/1 -> Sum/2
  Extract Bits2/1 -> Mux5/1
  Data Type Conversion5/1 -> Extract Bits2/1, Extract Bits3/1
  SPI WriteRead3/1 -> Terminator5/1
  Sum/1 -> Data Type Conversion5/1
  IL/1 -> Sum/1

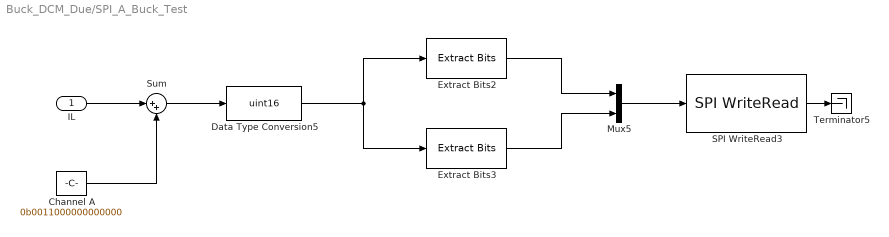
== system Buck_DCM_Due/SPI_A_Buck_Test ==
  IL : Inport
  Channel A : Constant  Value=0b0011000000000000
  Data Type Conversion5 : DataTypeConversion  OutDataTypeStr=uint16  RndMeth=Nearest
  Extract Bits2 : simulink/Logic and Bit Operations/Extract Bits  bitsToExtract=Range starting with most significant bit  numBits=8  bitIdxRange=[0 7]  outScalingMode=Treat bit field as an integer
  Extract Bits3 : simulink/Logic and Bit Operations/Extract Bits  bitsToExtract=Range ending with least significant bit  numBits=8  bitIdxRange=[0 7]  outScalingMode=Treat bit field as an integer
  Mux5 : Mux  Inputs=2
  SPI WriteRead3 : arduinolib/SPI WriteRead  slaveSelectPin_=4  blockPlatform=arduino
      settings: SourceProductBaseCode=ARDUINO
  Sum : Sum  Inputs=|++
  Terminator5 : Terminator
  wires:
  Extract Bits3/1 -> Mux5/2
  Mux5/1 -> SPI WriteRead3/1
  Channel A/1 -> Sum/2
  Extract Bits2/1 -> Mux5/1
  Data Type Conversion5/1 -> Extract Bits2/1, Extract Bits3/1
  SPI WriteRead3/1 -> Terminator5/1
  Sum/1 -> Data Type Conversion5/1
  IL/1 -> Sum/1

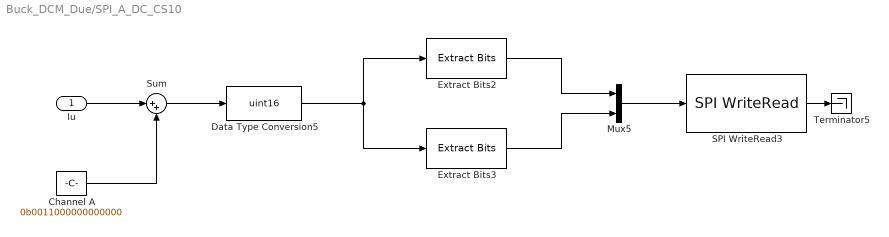
== system Buck_DCM_Due/SPI_A_DC_CS10 ==
  Iu : Inport
  Channel A : Constant  Value=0b0011000000000000
  Data Type Conversion5 : DataTypeConversion  OutDataTypeStr=uint16  RndMeth=Nearest
  Extract Bits2 : simulink/Logic and Bit Operations/Extract Bits  bitsToExtract=Range starting with most significant bit  numBits=8  bitIdxRange=[0 7]  outScalingMode=Treat bit field as an integer
  Extract Bits3 : simulink/Logic and Bit Operations/Extract Bits  bitsToExtract=Range ending with least significant bit  numBits=8  bitIdxRange=[0 7]  outScalingMode=Treat bit field as an integer
  Mux5 : Mux  Inputs=2
  SPI WriteRead3 : arduinolib/SPI WriteRead  slaveSelectPin_=10  blockPlatform=arduino
      settings: SourceProductBaseCode=ARDUINO
  Sum : Sum  Inputs=|++
  Terminator5 : Terminator
  wires:
  Extract Bits3/1 -> Mux5/2
  Mux5/1 -> SPI WriteRead3/1
  Channel A/1 -> Sum/2
  Extract Bits2/1 -> Mux5/1
  Data Type Conversion5/1 -> Extract Bits2/1, Extract Bits3/1
  SPI WriteRead3/1 -> Terminator5/1
  Sum/1 -> Data Type Conversion5/1
  Iu/1 -> Sum/1

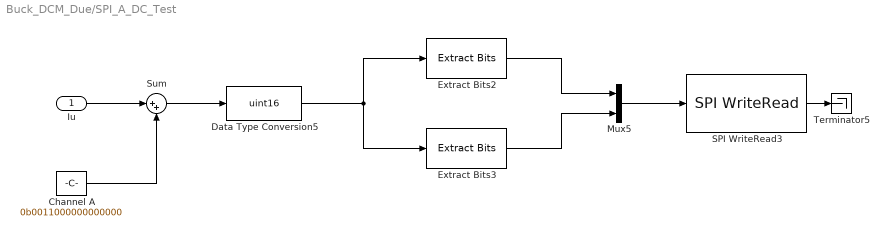
== system Buck_DCM_Due/SPI_A_DC_Test ==
  Iu : Inport
  Channel A : Constant  Value=0b0011000000000000  SampleTime=T
  Data Type Conversion5 : DataTypeConversion  OutDataTypeStr=uint16  RndMeth=Nearest
  Extract Bits2 : simulink/Logic and Bit Operations/Extract Bits  bitsToExtract=Range starting with most significant bit  numBits=8  bitIdxRange=[0 7]  outScalingMode=Treat bit field as an integer
  Extract Bits3 : simulink/Logic and Bit Operations/Extract Bits  bitsToExtract=Range ending with least significant bit  numBits=8  bitIdxRange=[0 7]  outScalingMode=Treat bit field as an integer
  Mux5 : Mux  Inputs=2
  SPI WriteRead3 : arduinolib/SPI WriteRead  slaveSelectPin_=10  blockPlatform=arduino
      settings: SourceProductBaseCode=ARDUINO
  Sum : Sum  Inputs=|++
  Terminator5 : Terminator
  wires:
  Extract Bits3/1 -> Mux5/2
  Mux5/1 -> SPI WriteRead3/1
  Channel A/1 -> Sum/2
  Extract Bits2/1 -> Mux5/1
  Data Type Conversion5/1 -> Extract Bits2/1, Extract Bits3/1
  SPI WriteRead3/1 -> Terminator5/1
  Sum/1 -> Data Type Conversion5/1
  Iu/1 -> Sum/1

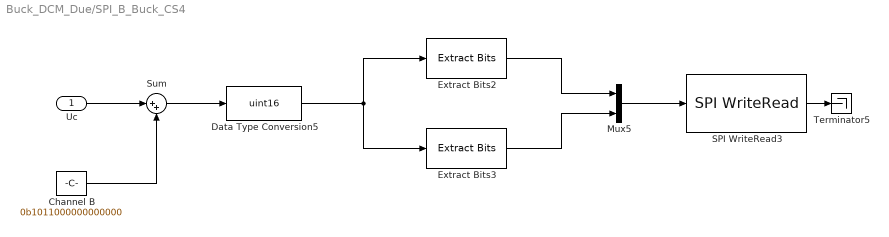
== system Buck_DCM_Due/SPI_B_Buck_CS4 ==
  Uc : Inport
  Channel B : Constant  Value=0b1011000000000000
  Data Type Conversion5 : DataTypeConversion  OutDataTypeStr=uint16  RndMeth=Nearest
  Extract Bits2 : simulink/Logic and Bit Operations/Extract Bits  bitsToExtract=Range starting with most significant bit  numBits=8  bitIdxRange=[0 7]  outScalingMode=Treat bit field as an integer
  Extract Bits3 : simulink/Logic and Bit Operations/Extract Bits  bitsToExtract=Range ending with least significant bit  numBits=8  bitIdxRange=[0 7]  outScalingMode=Treat bit field as an integer
  Mux5 : Mux  Inputs=2
  SPI WriteRead3 : arduinolib/SPI WriteRead  slaveSelectPin_=4  blockPlatform=arduino
      settings: SourceProductBaseCode=ARDUINO
  Sum : Sum  Inputs=|++
  Terminator5 : Terminator
  wires:
  Extract Bits3/1 -> Mux5/2
  Mux5/1 -> SPI WriteRead3/1
  Channel B/1 -> Sum/2
  Extract Bits2/1 -> Mux5/1
  Data Type Conversion5/1 -> Extract Bits2/1, Extract Bits3/1
  SPI WriteRead3/1 -> Terminator5/1
  Sum/1 -> Data Type Conversion5/1
  Uc/1 -> Sum/1

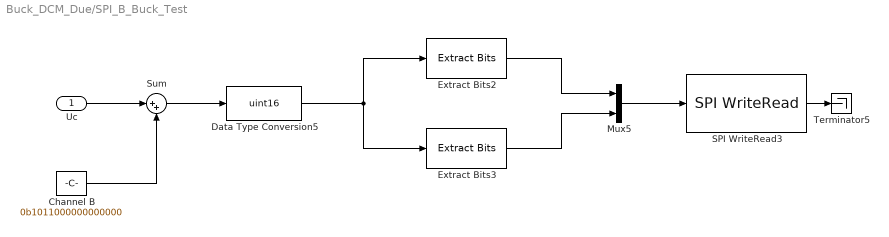
== system Buck_DCM_Due/SPI_B_Buck_Test ==
  Uc : Inport
  Channel B : Constant  Value=0b1011000000000000
  Data Type Conversion5 : DataTypeConversion  OutDataTypeStr=uint16  RndMeth=Nearest
  Extract Bits2 : simulink/Logic and Bit Operations/Extract Bits  bitsToExtract=Range starting with most significant bit  numBits=8  bitIdxRange=[0 7]  outScalingMode=Treat bit field as an integer
  Extract Bits3 : simulink/Logic and Bit Operations/Extract Bits  bitsToExtract=Range ending with least significant bit  numBits=8  bitIdxRange=[0 7]  outScalingMode=Treat bit field as an integer
  Mux5 : Mux  Inputs=2
  SPI WriteRead3 : arduinolib/SPI WriteRead  slaveSelectPin_=4  blockPlatform=arduino
      settings: SourceProductBaseCode=ARDUINO
  Sum : Sum  Inputs=|++
  Terminator5 : Terminator
  wires:
  Extract Bits3/1 -> Mux5/2
  Mux5/1 -> SPI WriteRead3/1
  Channel B/1 -> Sum/2
  Extract Bits2/1 -> Mux5/1
  Data Type Conversion5/1 -> Extract Bits2/1, Extract Bits3/1
  SPI WriteRead3/1 -> Terminator5/1
  Sum/1 -> Data Type Conversion5/1
  Uc/1 -> Sum/1

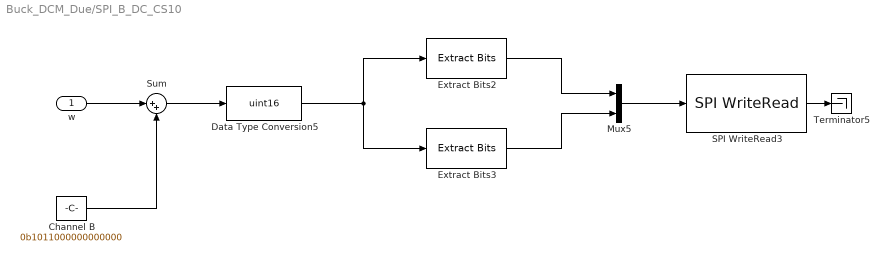
== system Buck_DCM_Due/SPI_B_DC_CS10 ==
  w : Inport
  Channel B : Constant  Value=0b1011000000000000
  Data Type Conversion5 : DataTypeConversion  OutDataTypeStr=uint16  RndMeth=Nearest
  Extract Bits2 : simulink/Logic and Bit Operations/Extract Bits  bitsToExtract=Range starting with most significant bit  numBits=8  bitIdxRange=[0 7]  outScalingMode=Treat bit field as an integer
  Extract Bits3 : simulink/Logic and Bit Operations/Extract Bits  bitsToExtract=Range ending with least significant bit  numBits=8  bitIdxRange=[0 7]  outScalingMode=Treat bit field as an integer
  Mux5 : Mux  Inputs=2
  SPI WriteRead3 : arduinolib/SPI WriteRead  slaveSelectPin_=10  blockPlatform=arduino
      settings: SourceProductBaseCode=ARDUINO
  Sum : Sum  Inputs=|++
  Terminator5 : Terminator
  wires:
  Extract Bits3/1 -> Mux5/2
  Mux5/1 -> SPI WriteRead3/1
  Channel B/1 -> Sum/2
  Extract Bits2/1 -> Mux5/1
  Data Type Conversion5/1 -> Extract Bits2/1, Extract Bits3/1
  SPI WriteRead3/1 -> Terminator5/1
  Sum/1 -> Data Type Conversion5/1
  w/1 -> Sum/1

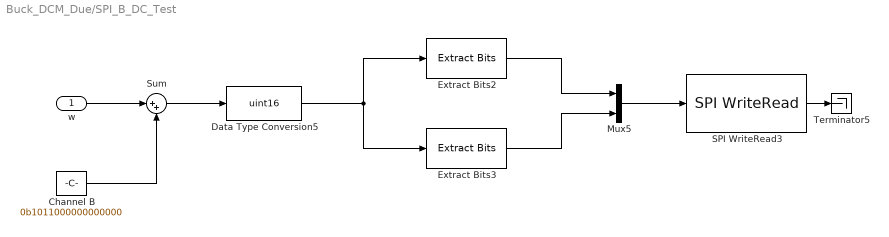
== system Buck_DCM_Due/SPI_B_DC_Test ==
  w : Inport
  Channel B : Constant  Value=0b1011000000000000  SampleTime=T
  Data Type Conversion5 : DataTypeConversion  OutDataTypeStr=uint16  RndMeth=Nearest
  Extract Bits2 : simulink/Logic and Bit Operations/Extract Bits  bitsToExtract=Range starting with most significant bit  numBits=8  bitIdxRange=[0 7]  outScalingMode=Treat bit field as an integer
  Extract Bits3 : simulink/Logic and Bit Operations/Extract Bits  bitsToExtract=Range ending with least significant bit  numBits=8  bitIdxRange=[0 7]  outScalingMode=Treat bit field as an integer
  Mux5 : Mux  Inputs=2
  SPI WriteRead3 : arduinolib/SPI WriteRead  slaveSelectPin_=10  blockPlatform=arduino
      settings: SourceProductBaseCode=ARDUINO
  Sum : Sum  Inputs=|++
  Terminator5 : Terminator
  wires:
  Extract Bits3/1 -> Mux5/2
  Mux5/1 -> SPI WriteRead3/1
  Channel B/1 -> Sum/2
  Extract Bits2/1 -> Mux5/1
  Data Type Conversion5/1 -> Extract Bits2/1, Extract Bits3/1
  SPI WriteRead3/1 -> Terminator5/1
  Sum/1 -> Data Type Conversion5/1
  w/1 -> Sum/1

== system Buck_DCM_Due/Speed Controller ==
  Mc : Inport
  w_mes : Inport  Port=2
  w_ref : Inport  Port=3
  P Controller : Gain  Gain=Kp_W
  Sum : Sum  Inputs=|++
  Sum1 : Sum  Inputs=|-+
  M_ref : Outport  InitialOutput=0  VectorParamsAs1DForOutWhenUnconnected=off
  wires:
  Sum/1 -> M_ref/1
  w_ref/1 -> Sum1/2
  Sum1/1 -> P Controller/1
  P Controller/1 -> Sum/2
  Mc/1 -> Sum/1
  w_mes/1 -> Sum1/1
